simulink model "REMUS_CONTROL_helix"  (R2018a)
settings: Solver=FixedStepAuto  StartTime=0.0  StopTime=800  FixedStep=0.01  RelTol=1e-3  EnableMultiTasking=on
libraries: simulink x5, dspstat3 x1, simulink_extras x1
settings Model: Creator=wariza  LastModifiedBy=wariza
settings SolverCC: ZeroCrossControl=EnableAll  ZeroCrossAlgorithm=Adaptive  SolverResetMethod=Robust  PositivePriorityOrder=on  AutoInsertRateTranBlk=on  InsertRTBMode=Always
settings DataIOCC: LimitDataPoints=on  SaveFormat=Array
settings OptimizationCC: LifeSpan=inf
settings DebuggingCC: SolverPrmCheckMsg=warning  SFUnexpectedBacktrackingDiag=warning  SFNoUnconditionalDefaultTransitionDiag=warning  SFExecutionAtInitializationDiag=none
settings HardwareCC: ProdBitPerPointer=32  ProdBitPerSizeT=32  ProdBitPerPtrDiffT=32  ProdLargestAtomicFloat=None  ProdIntDivRoundTo=Undefined  ProdEndianess=Unspecified  ProdWordSize=32  ProdHWDeviceType=32-bit Generic
settings ModelReferenceCC: PropagateSignalLabelsOutOfModel=off
settings CodeAppCC: StateflowObjectComments=on
settings GRTTargetCC: TargetLangStandard=C89/C90 (ANSI)  GeneratePreprocessorConditionals=Disable all
settings ConfigComp: CovMetricSettings=dw  CovHtmlReporting=on  CovSaveCumulativeToWorkspaceVar=on  CovSaveSingleToWorkspaceVar=on  CovExternalEMLEnable=off  CovSFcnEnable=off

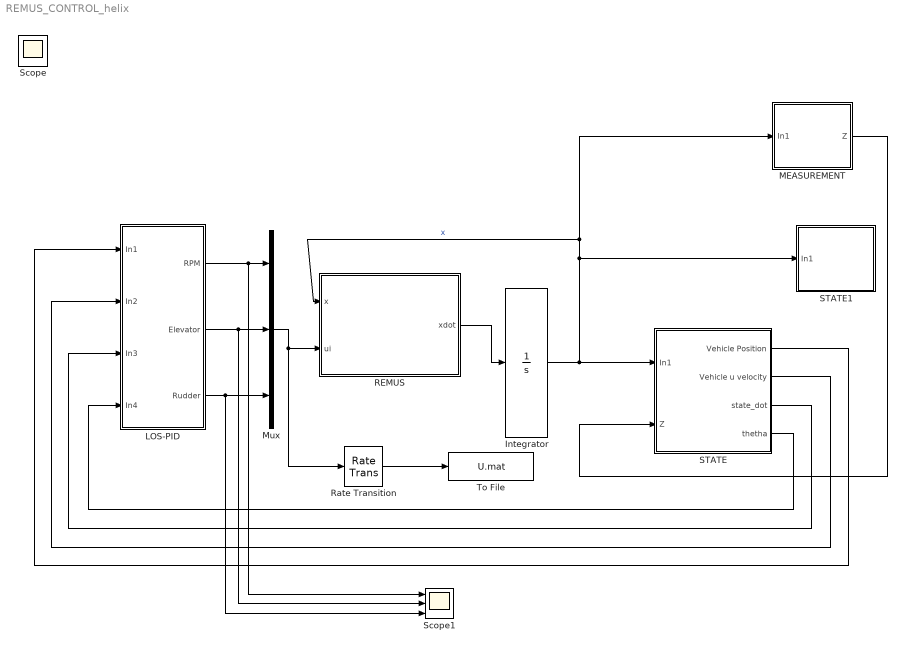
== system REMUS_CONTROL_helix ==
  Integrator : Integrator  InitialCondition=[0.5,0,0,0,0,0,60,3,0,0,0,3*pi/4]  ContinuousStateAttributes='position'
  LOS-PID : Subsystem
  MEASUREMENT : Subsystem
  Mux : Mux  Inputs=3
  REMUS : MATLAB Function  TreatAsAtomicUnit=on
  Rate Transition : RateTransition  OutPortSampleTime=0.01
  STATE : Subsystem
  STATE1 : Subsystem
  Scope1 : Scope  NumInputPorts=3
  To File : ToFile  Filename=U.mat  MatrixName=U
  Scope : Scope
  wires:
  Rate Transition/1 -> To File/1
  REMUS/1(xdot) -> Integrator/1
  Mux/1 -> Rate Transition/1, REMUS/2(ui)
  Integrator/1 -> STATE/1(In1), STATE1/1(In1), MEASUREMENT/1(In1), REMUS/1(x)  "x"
  MEASUREMENT/1(Z) -> STATE/2(Z)
  STATE/1(Vehicle Position) -> LOS-PID/1(In1)
  STATE/2(Vehicle u velocity) -> LOS-PID/2(In2)
  STATE/3(state_dot) -> LOS-PID/3(In3)
  STATE/4(thetha) -> LOS-PID/4(In4)
  LOS-PID/1(RPM) -> Scope1/1, Mux/1
  LOS-PID/2(Elevator) -> Scope1/2, Mux/2
  LOS-PID/3(Rudder) -> Scope1/3, Mux/3

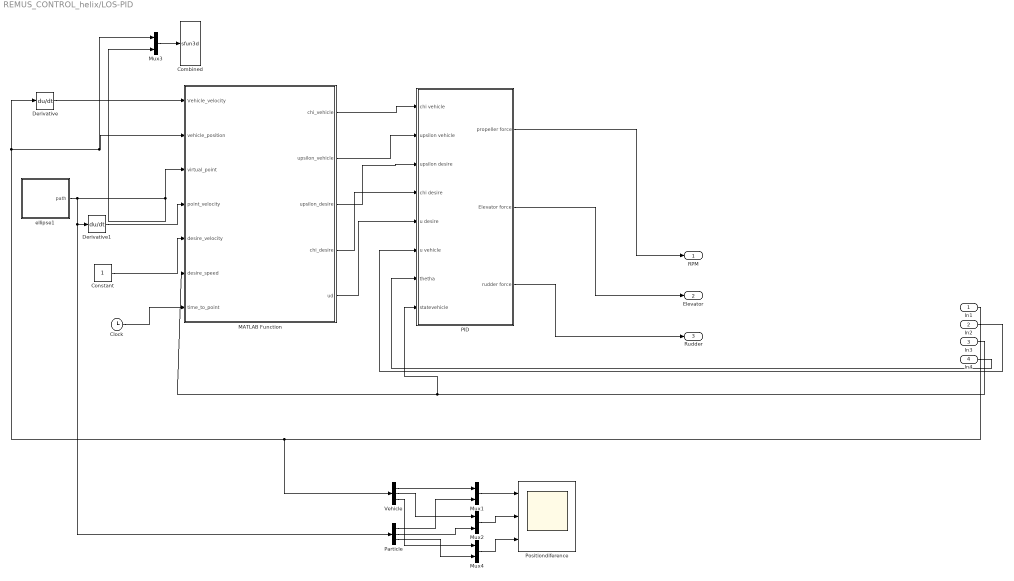
== system REMUS_CONTROL_helix/LOS-PID ==
  In1 : Inport
  In2 : Inport  Port=2
  In3 : Inport  Port=3
  In4 : Inport  Port=4
  Clock : Clock
  Combined : S-Function  LoadFcn=if exist('sfun3d','file'), sfun3d([],[],[],'LoadBlock'); end  FunctionName=sfun3d  Parameters=ax,T,np,cp,gd,ls,mk  SFunctionDeploymentMode=off  EnableBusSupport=off  mask(3D Graph){np=2, ax=[-100 100 -100 100 0 10], cp=[200 300 200], gd=on, ls=-, mk=none, T=-1}
      mask prompts: np "Number of point (lines)"; ax "[xmin xmax  ymin ymax zmin zmax]"; cp "Camera position (use [0 0 1] for 2D XY view)"; gd "Grid (on|off)"; ls "LineStyle"; mk "Marker"; T "Sampling Time"
      mask help:
      | This block plots the position of several points in the XYZ space. The input contains the coordinates of all the points (x1,y1,z1,x2,y2,z2,...).
      | The number of points (lines), the XYZ ranges, camera position, grid, linestyle, marker and sampling time, can be set as mask parameters.
      settings: CopyFcn=if exist('sfun3d','file'), sfun3d([],[],[],'CopyBlock'); end  DeleteFcn=if exist('sfun3d','file'), sfun3d([],[],[],'DeleteBlock'); end  NameChangeFcn=if exist('sfun3d','file'), sfun3d([],[],[],'NameChange'); end
      mask Help:
      | This block plots the position of several points in the XYZ space. The input contains the coordinates of all the points (x1,y1,z1,x2,y2,z2,...).
      | The number of points (lines), the XYZ ranges, camera position, grid, linestyle, marker and sampling time, can be set as mask parameters.
      mask TypeOptions ls: - | -- | : | -. | none
      mask TypeOptions mk: none | . | + | o | * | x | square | diamond | v | ^ | > | < | pentagram | hexagram
      mask Display: plot([.05 .95 .95 .05 .05],[.45 .45 .95 .95 .45], 0.5+cos(0:0.1:2*pi)*0.3,0.7+sin(0:0.1:2*pi)*0.2)
  Constant : Constant
  Derivative : Derivative
  Derivative1 : Derivative
  MATLAB Function : MATLAB Function  TreatAsAtomicUnit=on
  Mux{1..4} (4 alike) : Mux  Inputs=2
  PID : Subsystem
  Particle : Demux  Outputs=3
  Positiondiference : Scope  NumInputPorts=3
  Vehicle : Demux  Outputs=3
  ellipse1 : Subsystem
  RPM : Outport
  Elevator : Outport  Port=2
  Rudder : Outport  Port=3
  wires:
  Particle/2 -> Mux2/2
  Mux2/1 -> Positiondiference/2
  ellipse1/1(path) -> Derivative1/1, Particle/1, MATLAB Function/3(virtual_point), Mux3/2
  MATLAB Function/3(upsilon_desire) -> PID/3(upsilon desire)
  In4/1 -> PID/7(thetha)
  Particle/1 -> Mux1/2
  MATLAB Function/1(chi_vehicle) -> PID/1(chi vehicle)
  Mux3/1 -> Combined/1
  In1/1 -> Vehicle/1, Derivative/1, Mux3/1, MATLAB Function/2(vehicle_position)
  Mux1/1 -> Positiondiference/1
  MATLAB Function/2(upsilon_vehicle) -> PID/2(upsilon vehicle)
  Constant/1 -> MATLAB Function/5(desire_velocity)
  Mux4/1 -> Positiondiference/3
  PID/1(propeller force) -> RPM/1
  Clock/1 -> MATLAB Function/7(time_to_point)
  Derivative/1 -> MATLAB Function/1(Vehicle_velocity)
  Vehicle/2 -> Mux2/1
  Vehicle/3 -> Mux4/1
  Particle/3 -> Mux4/2
  PID/3(rudder force) -> Rudder/1
  MATLAB Function/5(ud) -> PID/5(u desire)
  In3/1 -> PID/8(statevehicle), MATLAB Function/6(desire_speed)
  Derivative1/1 -> MATLAB Function/4(point_velocity)
  MATLAB Function/4(chi_desire) -> PID/4(chi desire)
  Vehicle/1 -> Mux1/1
  In2/1 -> PID/6(u vehicle)
  PID/2(Elevator force) -> Elevator/1

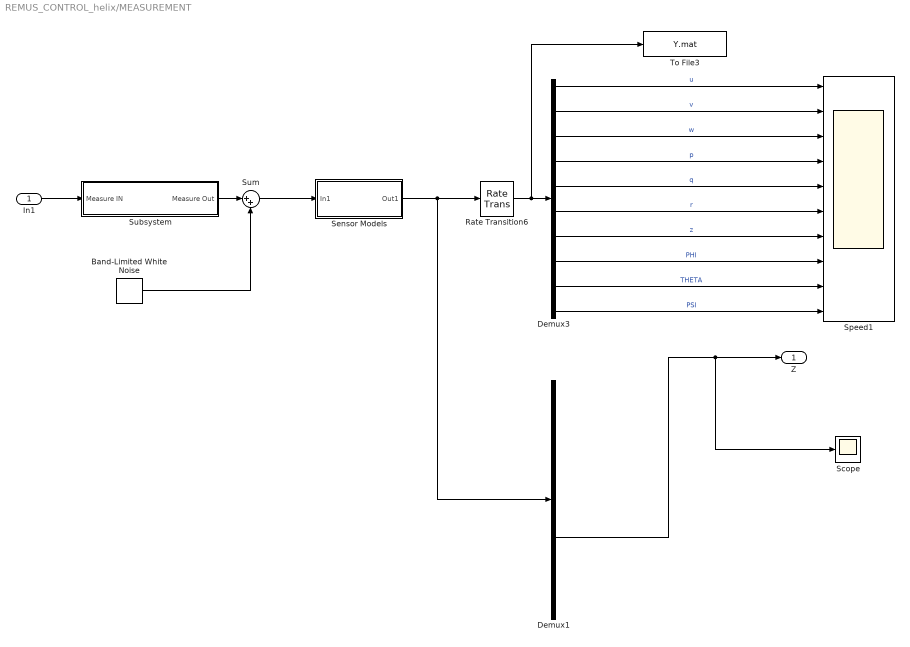
== system REMUS_CONTROL_helix/MEASUREMENT ==
  In1 : Inport
  Band-Limited White Noise : simulink/Sources/Band-Limited White Noise  Cov=[3e-8;2e-7;1e-8;1e-8;1e-7;1e-7;0.0000001;1e-9;1e-7;1e-5]  Ts=0.1  seed=[1;2;3;4;5;6;9;10;11;12]  VectorParams1D=off
  Demux1 : Demux  Outputs=10
  Demux3 : Demux  Outputs=10
  Rate Transition6 : RateTransition  OutPortSampleTime=0.01
  Scope : Scope
  Sensor Models : Subsystem
  Speed1 : Scope  NumInputPorts=10
  Subsystem : Subsystem
  Sum : Sum  Inputs=|++
  To File3 : ToFile  Filename=Y.mat  MatrixName=Y
  Z : Outport
  wires:
  Subsystem/1(Measure Out) -> Sum/1
  Demux3/3 -> Speed1/3  "w"
  Band-Limited White Noise/1 -> Sum/2
  Rate Transition6/1 -> To File3/1, Demux3/1
  Demux3/4 -> Speed1/4  "p"
  Demux3/2 -> Speed1/2  "v"
  Demux3/1 -> Speed1/1  "u"
  Sum/1 -> Sensor Models/1(In1)
  Demux3/5 -> Speed1/5  "q"
  Demux3/6 -> Speed1/6  "r"
  Demux3/9 -> Speed1/9  "THETA"
  Demux3/8 -> Speed1/8  "PHI"
  In1/1 -> Subsystem/1(Measure IN)
  Demux3/10 -> Speed1/10  "PSI"
  Demux3/7 -> Speed1/7  "z"
  Sensor Models/1(Out1) -> Demux1/1, Rate Transition6/1
  Demux1/7 -> Scope/1, Z/1

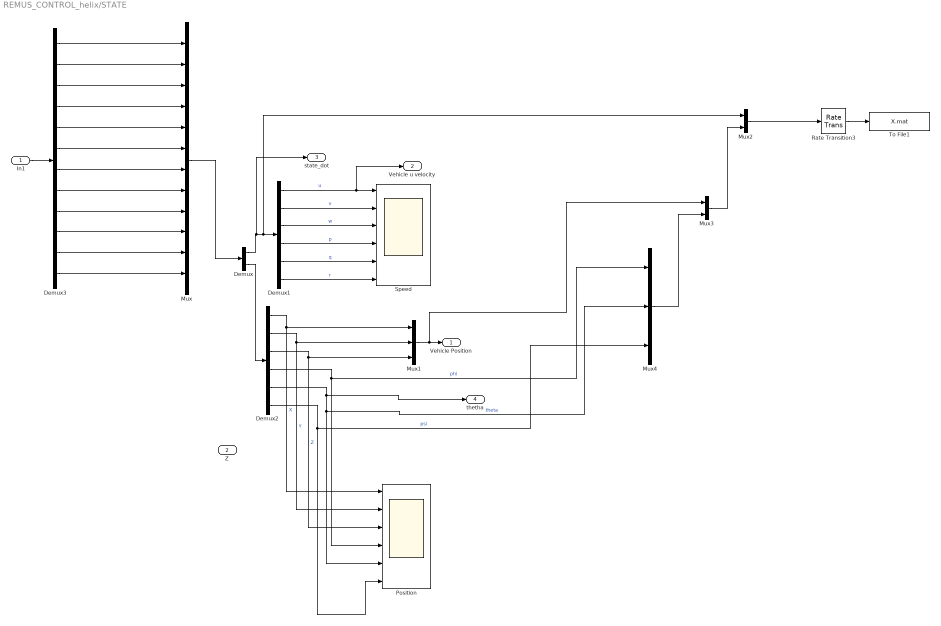
== system REMUS_CONTROL_helix/STATE ==
  In1 : Inport
  Z : Inport  Port=2
  Demux : Demux  Outputs=2
  Demux1 : Demux  Outputs=6
  Demux2 : Demux  Outputs=6
  Demux3 : Demux  Outputs=12
  Mux : Mux  Inputs=12
  Mux1 : Mux  Inputs=3
  Mux2 : Mux  Inputs=2
  Mux3 : Mux  Inputs=2
  Mux4 : Mux  Inputs=3
  Position : Scope  NumInputPorts=6
  Rate Transition3 : RateTransition  OutPortSampleTime=0.01
  Speed : Scope  NumInputPorts=6
  To File1 : ToFile  Filename=X.mat  MatrixName=X
  Vehicle Position : Outport
  Vehicle u velocity : Outport  Port=2
  state_dot : Outport  Port=3
  thetha : Outport  Port=4
  wires:
  Demux1/1 -> Vehicle u velocity/1, Speed/1  "u"
  Demux/2 -> Demux2/1
  Demux1/2 -> Speed/2  "v"
  Demux1/3 -> Speed/3  "w"
  Demux2/3 -> Mux1/3, Position/3  "Z"
  Demux2/5 -> thetha/1, Mux4/2, Position/5  "theta"
  Demux1/4 -> Speed/4  "p"
  Demux1/6 -> Speed/6  "r"
  Demux2/1 -> Mux1/1, Position/1  "X"
  Demux1/5 -> Speed/5  "q"
  Demux2/4 -> Mux4/1, Position/4  "phi"
  Demux2/2 -> Mux1/2, Position/2  "Y"
  Demux/1 -> state_dot/1, Mux2/1, Demux1/1
  Demux2/6 -> Mux4/3, Position/6  "psi"
  In1/1 -> Demux3/1
  Demux3/9 -> Mux/9
  Demux3/8 -> Mux/8
  Demux3/7 -> Mux/7
  Demux3/6 -> Mux/6
  Demux3/5 -> Mux/5
  Demux3/4 -> Mux/4
  Demux3/3 -> Mux/3
  Demux3/2 -> Mux/2
  Demux3/1 -> Mux/1
  Mux/1 -> Demux/1
  Mux1/1 -> Mux3/1, Vehicle Position/1
  Demux3/10 -> Mux/10
  Demux3/11 -> Mux/11
  Demux3/12 -> Mux/12
  Rate Transition3/1 -> To File1/1
  Mux2/1 -> Rate Transition3/1
  Mux4/1 -> Mux3/2
  Mux3/1 -> Mux2/2

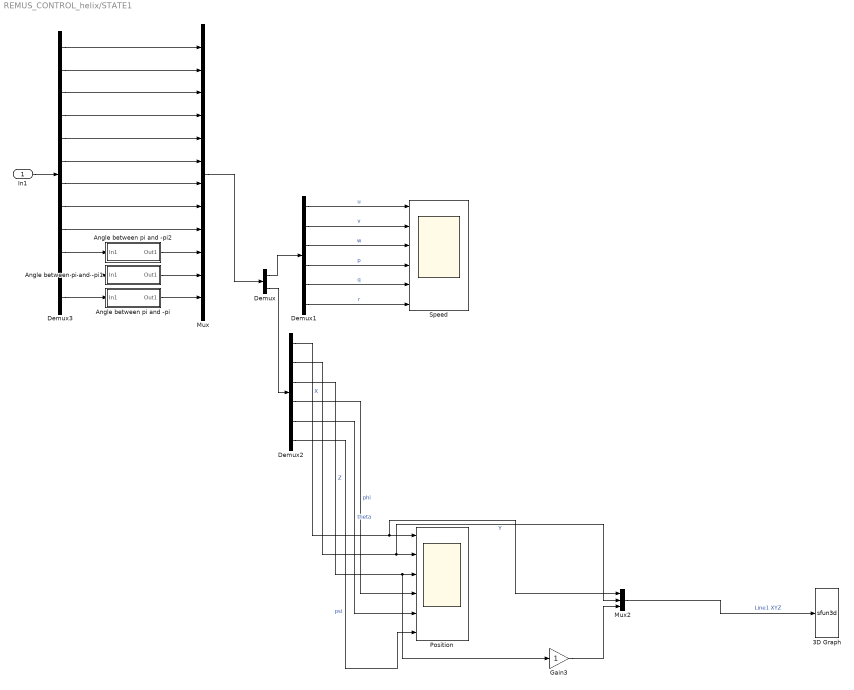
== system REMUS_CONTROL_helix/STATE1 ==
  In1 : Inport
  3D Graph : S-Function  LoadFcn=if exist('sfun3d','file'), sfun3d([],[],[],'LoadBlock'); end  FunctionName=sfun3d  Parameters=ax,T,np,cp,gd,ls,mk  SFunctionDeploymentMode=off  EnableBusSupport=off  mask(3D Graph){np=1, ax=[-100 100 -100 100 -30 30], cp=[20 40 20], gd=off, ls=-, mk=none, T=-1}
      mask prompts: np "Number of point (lines)"; ax "[xmin xmax  ymin ymax zmin zmax]"; cp "Camera position (use [0 0 1] for 2D XY view)"; gd "Grid (on|off)"; ls "LineStyle"; mk "Marker"; T "Sampling Time"
      mask help:
      | This block plots the position of several points in the XYZ space. The input contains the coordinates of all the points (x1,y1,z1,x2,y2,z2,...).
      | The number of points (lines), the XYZ ranges, camera position, grid, linestyle, marker and sampling time, can be set as mask parameters.
      settings: CopyFcn=if exist('sfun3d','file'), sfun3d([],[],[],'CopyBlock'); end  DeleteFcn=if exist('sfun3d','file'), sfun3d([],[],[],'DeleteBlock'); end  NameChangeFcn=if exist('sfun3d','file'), sfun3d([],[],[],'NameChange'); end
      mask Help:
      | This block plots the position of several points in the XYZ space. The input contains the coordinates of all the points (x1,y1,z1,x2,y2,z2,...).
      | The number of points (lines), the XYZ ranges, camera position, grid, linestyle, marker and sampling time, can be set as mask parameters.
      mask TypeOptions ls: - | -- | : | -. | none
      mask TypeOptions mk: none | . | + | o | * | x | square | diamond | v | ^ | > | < | pentagram | hexagram
      mask Display: plot([.05 .95 .95 .05 .05],[.45 .45 .95 .95 .45], 0.5+cos(0:0.1:2*pi)*0.3,0.7+sin(0:0.1:2*pi)*0.2)
  Angle between pi and -pi : Subsystem
  Angle between pi and -pi1 : Subsystem
  Angle between pi and -pi2 : Subsystem
  Demux : Demux  Outputs=2
  Demux1 : Demux  Outputs=6
  Demux2 : Demux  Outputs=6
  Demux3 : Demux  Outputs=12
  Gain3 : Gain
  Mux : Mux  Inputs=12
  Mux2 : Mux  Inputs=3
  Position : Scope  NumInputPorts=6
  Speed : Scope  NumInputPorts=6
  wires:
  Mux2/1 -> 3D Graph/1  "Line1 XYZ"
  Gain3/1 -> Mux2/3
  Demux1/1 -> Speed/1  "u"
  Demux/2 -> Demux2/1
  Demux1/2 -> Speed/2  "v"
  Demux1/3 -> Speed/3  "w"
  Demux2/3 -> Gain3/1, Position/3  "Z"
  Demux2/5 -> Position/5  "theta"
  Demux1/4 -> Speed/4  "p"
  Demux1/6 -> Speed/6  "r"
  Demux2/1 -> Mux2/1, Position/1  "X"
  Demux1/5 -> Speed/5  "q"
  Demux2/4 -> Position/4  "phi"
  Demux2/2 -> Mux2/2, Position/2  "Y"
  Demux/1 -> Demux1/1
  Demux2/6 -> Position/6  "psi"
  In1/1 -> Demux3/1
  Angle between pi and -pi/1(Out1) -> Mux/12
  Demux3/12 -> Angle between pi and -pi/1(In1)
  Angle between pi and -pi1/1(Out1) -> Mux/11
  Demux3/11 -> Angle between pi and -pi1/1(In1)
  Angle between pi and -pi2/1(Out1) -> Mux/10
  Demux3/10 -> Angle between pi and -pi2/1(In1)
  Demux3/9 -> Mux/9
  Demux3/8 -> Mux/8
  Demux3/7 -> Mux/7
  Demux3/6 -> Mux/6
  Demux3/5 -> Mux/5
  Demux3/4 -> Mux/4
  Demux3/3 -> Mux/3
  Demux3/2 -> Mux/2
  Demux3/1 -> Mux/1
  Mux/1 -> Demux/1

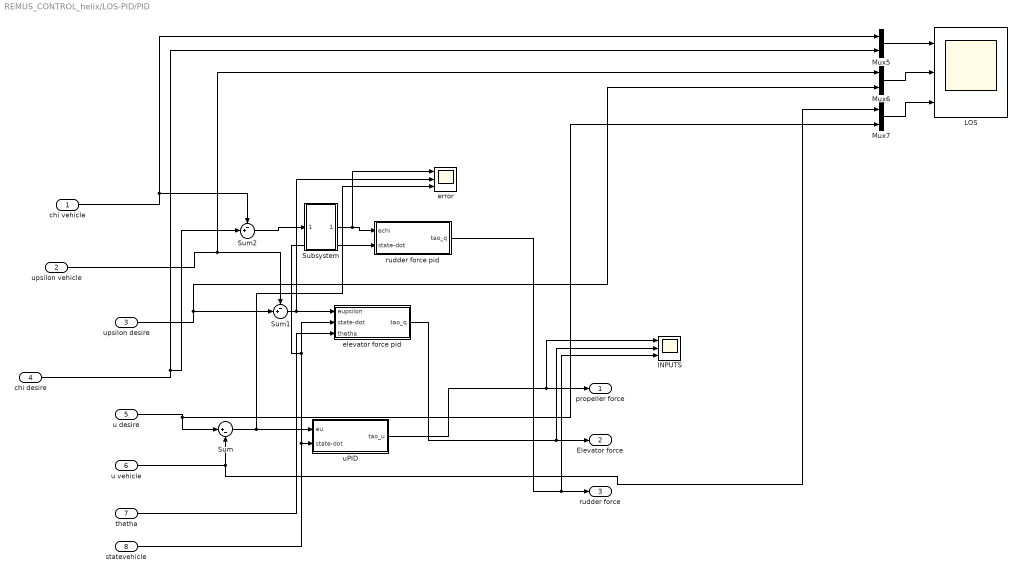
== system REMUS_CONTROL_helix/LOS-PID/PID ==
  chi vehicle : Inport
  upsilon vehicle : Inport  Port=2
  upsilon desire : Inport  Port=3
  chi desire : Inport  Port=4
  u desire : Inport  Port=5
  u vehicle : Inport  Port=6
  thetha : Inport  Port=7
  statevehicle : Inport  Port=8
  INPUTS : Scope  NumInputPorts=3
  LOS : Scope  NumInputPorts=3
  Mux5 : Mux  Inputs=2
  Mux6 : Mux  Inputs=2
  Mux7 : Mux  Inputs=2
  Subsystem : Subsystem
  Sum : Sum  Inputs=|+-
  Sum1 : Sum  Inputs=-+|
  Sum2 : Sum  Inputs=-+|
  elevator force pid : Subsystem
  error : Scope  NumInputPorts=3
  rudder force pid : Subsystem
  uPID : Subsystem
  propeller force : Outport
  Elevator force : Outport  Port=2
  rudder force : Outport  Port=3
  wires:
  uPID/1(tao_u) -> propeller force/1, INPUTS/1
  Mux6/1 -> LOS/2
  chi vehicle/1 -> Mux5/1, Sum2/1
  Sum/1 -> error/3, uPID/1(eu)
  statevehicle/1 -> rudder force pid/2(state-dot), elevator force pid/2(state-dot), uPID/2(state-dot)
  Sum1/1 -> error/2, elevator force pid/1(eupsilon)
  chi desire/1 -> Mux5/2, Sum2/2
  u vehicle/1 -> Mux7/1, Sum/2
  u desire/1 -> Sum/1, Mux7/2
  elevator force pid/1(tao_q) -> Elevator force/1, INPUTS/2
  rudder force pid/1(tao_q) -> rudder force/1, INPUTS/3
  upsilon desire/1 -> Mux6/2, Sum1/2
  Mux7/1 -> LOS/3
  thetha/1 -> elevator force pid/3(thetha)
  Mux5/1 -> LOS/1
  upsilon vehicle/1 -> Mux6/1, Sum1/1
  Sum2/1 -> Subsystem/1(In1)
  Subsystem/1(Out1) -> error/1, rudder force pid/1(echi)

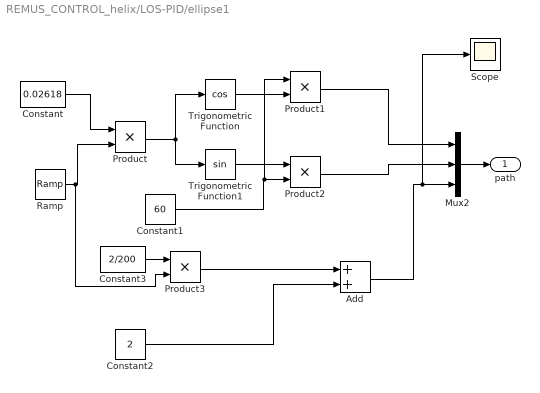
== system REMUS_CONTROL_helix/LOS-PID/ellipse1 ==
  Add : Sum
  Constant : Constant  Value=0.02618
  Constant1 : Constant  Value=60
  Constant2 : Constant  Value=2
  Constant3 : Constant  Value=2/200
  Mux2 : Mux  Inputs=3
  Product{,1..3} (4 alike) : Product
  Ramp : simulink/Sources/Ramp  slope=0.9  start=0  InitialOutput=0
  Scope : Scope
  Trigonometric Function : Trigonometry  Operator=cos
  Trigonometric Function1 : Trigonometry
  path : Outport
  wires:
  Mux2/1 -> path/1
  Ramp/1 -> Product3/2, Product/2
  Constant/1 -> Product/1
  Product/1 -> Trigonometric Function/1, Trigonometric Function1/1
  Trigonometric Function/1 -> Product1/2
  Trigonometric Function1/1 -> Product2/1
  Constant1/1 -> Product1/1, Product2/2
  Product1/1 -> Mux2/1
  Product2/1 -> Mux2/2
  Add/1 -> Scope/1, Mux2/3
  Constant2/1 -> Add/2
  Constant3/1 -> Product3/1
  Product3/1 -> Add/1

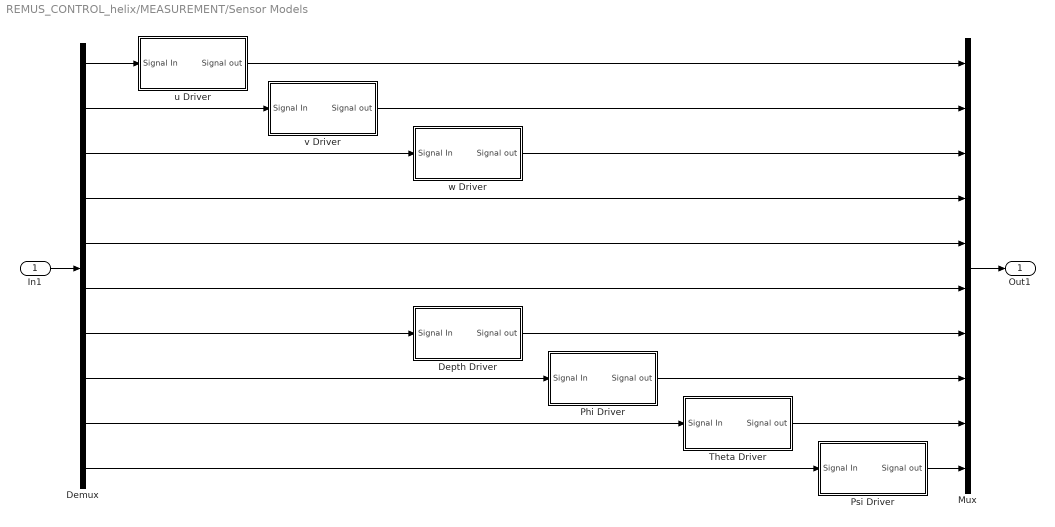
== system REMUS_CONTROL_helix/MEASUREMENT/Sensor Models ==
  In1 : Inport
  Demux : Demux  Outputs=10
  Depth Driver : Subsystem
  Mux : Mux  Inputs=10
  Phi Driver : Subsystem
  Psi Driver : Subsystem
  Theta Driver : Subsystem
  u Driver : Subsystem
  v Driver : Subsystem
  w Driver : Subsystem
  Out1 : Outport
  wires:
  In1/1 -> Demux/1
  Mux/1 -> Out1/1
  Demux/1 -> u Driver/1(Signal In)
  Demux/2 -> v Driver/1(Signal In)
  Demux/3 -> w Driver/1(Signal In)
  Demux/4 -> Mux/4
  Demux/5 -> Mux/5
  Demux/6 -> Mux/6
  Demux/8 -> Phi Driver/1(Signal In)
  Demux/9 -> Theta Driver/1(Signal In)
  Demux/10 -> Psi Driver/1(Signal In)
  Demux/7 -> Depth Driver/1(Signal In)
  Depth Driver/1(Signal out) -> Mux/7
  Phi Driver/1(Signal out) -> Mux/8
  Theta Driver/1(Signal out) -> Mux/9
  Psi Driver/1(Signal out) -> Mux/10
  u Driver/1(Signal out) -> Mux/1
  v Driver/1(Signal out) -> Mux/2
  w Driver/1(Signal out) -> Mux/3

== system REMUS_CONTROL_helix/MEASUREMENT/Subsystem ==
  note: u,v,w,p,q,r,Z,phi,theta,psi
  Measure IN : Inport
  Demux : Demux  Outputs=2
  Demux1 : Demux  Outputs=6
  Mux : Mux  Inputs=2
  Mux1 : Mux
  Measure Out : Outport
  wires:
  Measure IN/1 -> Demux/1
  Mux/1 -> Measure Out/1
  Demux/1 -> Mux/1
  Demux/2 -> Demux1/1
  Demux1/6 -> Mux1/4
  Demux1/5 -> Mux1/3
  Demux1/4 -> Mux1/2
  Demux1/3 -> Mux1/1
  Mux1/1 -> Mux/2

== system REMUS_CONTROL_helix/STATE1/Angle between pi and -pi ==
  In1 : Inport
  Atan2 : Trigonometry  Operator=atan2
  Cos : Trigonometry
  Sin : Trigonometry  Operator=cos
  Out1 : Outport
  wires:
  Cos/1 -> Atan2/1
  In1/1 -> Cos/1, Sin/1
  Sin/1 -> Atan2/2
  Atan2/1 -> Out1/1

== system REMUS_CONTROL_helix/STATE1/Angle between pi and -pi1 ==
  In1 : Inport
  Atan2 : Trigonometry  Operator=atan2
  Cos : Trigonometry
  Sin : Trigonometry  Operator=cos
  Out1 : Outport
  wires:
  Cos/1 -> Atan2/1
  In1/1 -> Cos/1, Sin/1
  Sin/1 -> Atan2/2
  Atan2/1 -> Out1/1

== system REMUS_CONTROL_helix/STATE1/Angle between pi and -pi2 ==
  In1 : Inport
  Atan2 : Trigonometry  Operator=atan2
  Cos : Trigonometry
  Sin : Trigonometry  Operator=cos
  Out1 : Outport
  wires:
  Cos/1 -> Atan2/1
  In1/1 -> Cos/1, Sin/1
  Sin/1 -> Atan2/2
  Atan2/1 -> Out1/1

== system REMUS_CONTROL_helix/LOS-PID/PID/Subsystem ==
  In1 : Inport
  Trigonometric Function : Trigonometry
  Trigonometric Function1 : Trigonometry  Operator=cos
  Trigonometric Function2 : Trigonometry  Operator=atan2
  Out1 : Outport
  wires:
  Trigonometric Function/1 -> Trigonometric Function2/1
  Trigonometric Function2/1 -> Out1/1
  In1/1 -> Trigonometric Function1/1, Trigonometric Function/1
  Trigonometric Function1/1 -> Trigonometric Function2/2

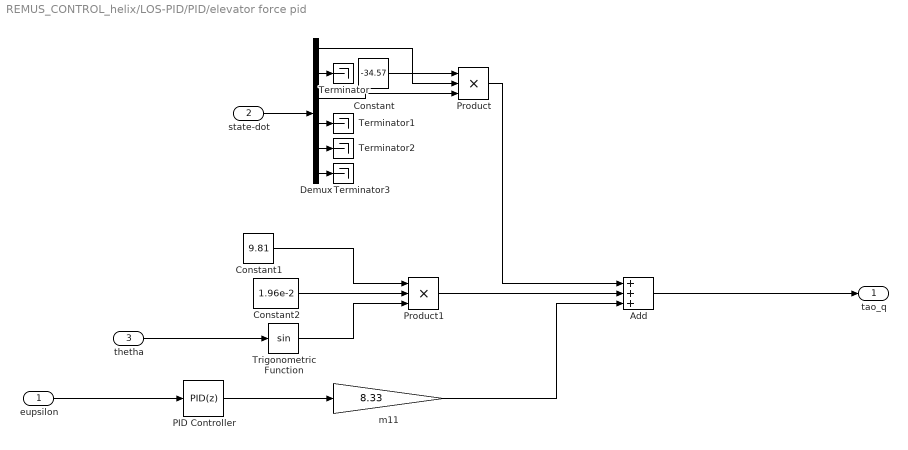
== system REMUS_CONTROL_helix/LOS-PID/PID/elevator force pid ==
  eupsilon : Inport
  state-dot : Inport  Port=2
  thetha : Inport  Port=3
  Add : Sum  Inputs=+++
  Constant : Constant  Value=-34.57
  Constant1 : Constant  Value=9.81
  Constant2 : Constant  Value=1.96e-2
  Demux : Demux  Outputs=6
  PID Controller : simulink/Continuous/PID Controller  Controller=PID  TimeDomain=Discrete-time  SampleTime=.4  IntegratorMethod=Forward Euler  FilterMethod=Forward Euler  Form=Parallel  UseFilter=off  ControllerParametersSource=internal  P=2  I=0  D=0.5  N=100  InitialConditionSource=internal  InitialConditionForIntegrator=0  InitialConditionForFilter=0  ExternalReset=none  LimitOutput=off  UpperSaturationLimit=inf  LowerSaturationLimit=-inf  LinearizeAsGain=on  AntiWindupMode=none  Kb=1  TrackingMode=off  Kt=1  PParamMin=[]  PParamMax=[]  IParamMin=[]  IParamMax=[]  DParamMin=[]  DParamMax=[]  NParamMin=[]  NParamMax=[]  KbParamMin=[]  KbParamMax=[]  KtParamMin=[]  KtParamMax=[]  POutMin=[]  POutMax=[]  IOutMin=[]  IOutMax=[]  DOutMin=[]  DOutMax=[]  NOutMin=[]  NOutMax=[]  KbOutMin=[]  KbOutMax=[]  KtOutMin=[]  KtOutMax=[]  IntegratorOutMin=[]  IntegratorOutMax=[]  FilterOutMin=[]  FilterOutMax=[]  SumOutMin=[]  SumOutMax=[]  SumI1OutMin=[]  SumI1OutMax=[]  SumI2OutMin=[]  SumI2OutMax=[]  SumI3OutMin=[]  SumI3OutMax=[]  SumDOutMin=[]  SumDOutMax=[]  SaturationOutMin=[]  SaturationOutMax=[]  IntegratorContinuousStateAttributes=''  IntegratorStateMustResolveToSignalObject=off  IntegratorRTWStateStorageClass=Auto  FilterContinuousStateAttributes=''  FilterStateMustResolveToSignalObject=off  FilterRTWStateStorageClass=Auto  DifferentiatorICPrevScaledInput=0  DifferentiatorOutMin=[]  DifferentiatorOutMax=[]  FilterDiffOutCoefMin=[]  FilterDiffOutCoefMax=[]  SumDenOutMin=[]  SumDenOutMax=[]  SumNumOutMin=[]  SumNumOutMax=[]  ReciprocalOutMin=[]  ReciprocalOutMax=[]  DivideOutMin=[]  DivideOutMax=[]  TunerSelectOption=Transfer Function Based (PID Tuner App)
  Product : Product  Inputs=3
  Product1 : Product  Inputs=3
  Terminator{,1..3} (4 alike) : Terminator
  Trigonometric Function : Trigonometry
  m11 : Gain  Gain=8.33
  tao_q : Outport  InitialOutput=0
  wires:
  state-dot/1 -> Demux/1
  Constant/1 -> Product/1
  m11/1 -> Add/3
  Constant1/1 -> Product1/1
  Demux/1 -> Product/2
  Demux/3 -> Product/3
  Product/1 -> Add/1
  Constant2/1 -> Product1/2
  Trigonometric Function/1 -> Product1/3
  Product1/1 -> Add/2
  thetha/1 -> Trigonometric Function/1
  PID Controller/1 -> m11/1
  eupsilon/1 -> PID Controller/1
  Add/1 -> tao_q/1
  Demux/6 -> Terminator3/1
  Demux/5 -> Terminator2/1
  Demux/4 -> Terminator1/1
  Demux/2 -> Terminator/1

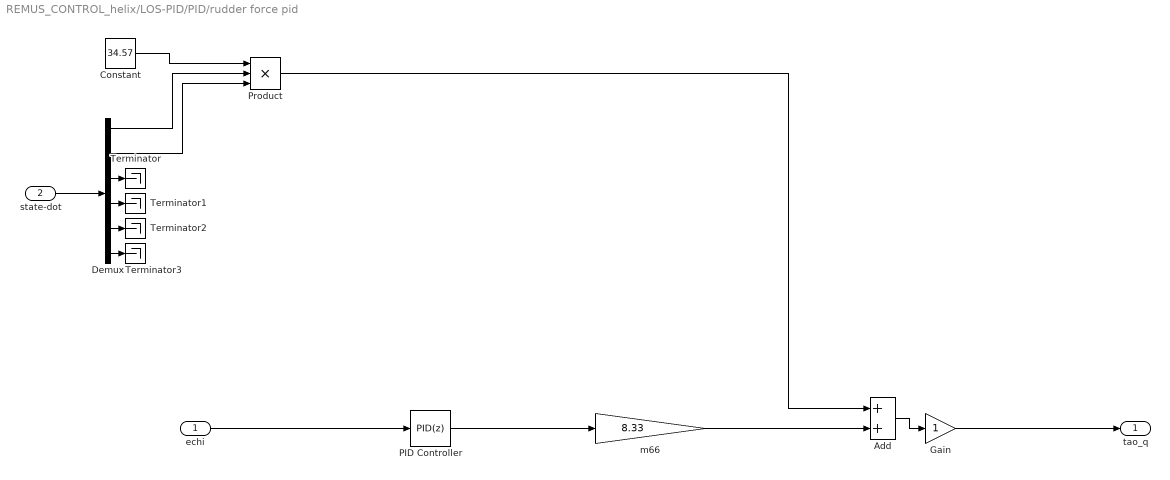
== system REMUS_CONTROL_helix/LOS-PID/PID/rudder force pid ==
  echi : Inport
  state-dot : Inport  Port=2
  Add : Sum
  Constant : Constant  Value=34.57
  Demux : Demux  Outputs=6
  Gain : Gain
  PID Controller : simulink/Continuous/PID Controller  Controller=PID  TimeDomain=Discrete-time  SampleTime=0.4  IntegratorMethod=Forward Euler  FilterMethod=Forward Euler  Form=Parallel  UseFilter=off  ControllerParametersSource=internal  P=3  I=0  D=1  N=100  InitialConditionSource=internal  InitialConditionForIntegrator=0  InitialConditionForFilter=0  ExternalReset=none  LimitOutput=on  UpperSaturationLimit=inf  LowerSaturationLimit=-inf  LinearizeAsGain=on  AntiWindupMode=clamping  Kb=1  TrackingMode=off  Kt=1  PParamMin=[]  PParamMax=[]  IParamMin=[]  IParamMax=[]  DParamMin=[]  DParamMax=[]  NParamMin=[]  NParamMax=[]  KbParamMin=[]  KbParamMax=[]  KtParamMin=[]  KtParamMax=[]  POutMin=[]  POutMax=[]  IOutMin=[]  IOutMax=[]  DOutMin=[]  DOutMax=[]  NOutMin=[]  NOutMax=[]  KbOutMin=[]  KbOutMax=[]  KtOutMin=[]  KtOutMax=[]  IntegratorOutMin=[]  IntegratorOutMax=[]  FilterOutMin=[]  FilterOutMax=[]  SumOutMin=[]  SumOutMax=[]  SumI1OutMin=[]  SumI1OutMax=[]  SumI2OutMin=[]  SumI2OutMax=[]  SumI3OutMin=[]  SumI3OutMax=[]  SumDOutMin=[]  SumDOutMax=[]  SaturationOutMin=[]  SaturationOutMax=[]  IntegratorContinuousStateAttributes=''  IntegratorStateMustResolveToSignalObject=off  IntegratorRTWStateStorageClass=Auto  FilterContinuousStateAttributes=''  FilterStateMustResolveToSignalObject=off  FilterRTWStateStorageClass=Auto  DifferentiatorICPrevScaledInput=0  DifferentiatorOutMin=[]  DifferentiatorOutMax=[]  FilterDiffOutCoefMin=[]  FilterDiffOutCoefMax=[]  SumDenOutMin=[]  SumDenOutMax=[]  SumNumOutMin=[]  SumNumOutMax=[]  ReciprocalOutMin=[]  ReciprocalOutMax=[]  DivideOutMin=[]  DivideOutMax=[]  TunerSelectOption=Transfer Function Based (PID Tuner App)
  Product : Product  Inputs=3
  Terminator{,1..3} (4 alike) : Terminator
  m66 : Gain  Gain=8.33
  tao_q : Outport  InitialOutput=0
  wires:
  state-dot/1 -> Demux/1
  Constant/1 -> Product/1
  m66/1 -> Add/2
  Demux/1 -> Product/2
  Product/1 -> Add/1
  Demux/2 -> Product/3
  Add/1 -> Gain/1
  PID Controller/1 -> m66/1
  Gain/1 -> tao_q/1
  Demux/6 -> Terminator3/1
  Demux/5 -> Terminator2/1
  Demux/4 -> Terminator1/1
  Demux/3 -> Terminator/1
  echi/1 -> PID Controller/1

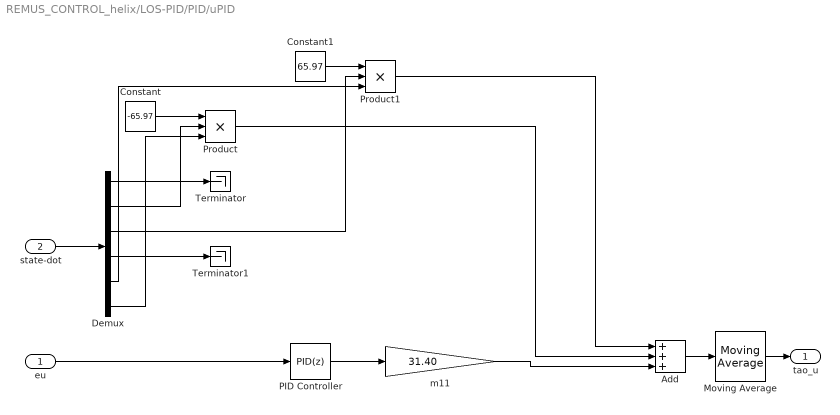
== system REMUS_CONTROL_helix/LOS-PID/PID/uPID ==
  eu : Inport
  state-dot : Inport  Port=2
  Add : Sum  Inputs=+++
  Constant : Constant  Value=-65.97
  Constant1 : Constant  Value=65.97
  Demux : Demux  Outputs=6
  Moving Average : dspstat3/Moving Average  Method=Exponential weighting  ForgettingFactorPort=off  SpecifyWindowLength=on  WindowLength=20  ForgettingFactor=0.9  SimulateUsing=Code generation
  PID Controller : simulink/Continuous/PID Controller  Controller=PID  TimeDomain=Discrete-time  SampleTime=0.4  IntegratorMethod=Forward Euler  FilterMethod=Forward Euler  Form=Parallel  UseFilter=off  ControllerParametersSource=internal  P=100  I=1  D=2  N=50  InitialConditionSource=internal  InitialConditionForIntegrator=0  InitialConditionForFilter=0  ExternalReset=none  ZeroCross=off  LimitOutput=off  UpperSaturationLimit=inf  LowerSaturationLimit=-inf  LinearizeAsGain=on  AntiWindupMode=none  Kb=1  TrackingMode=off  Kt=1  PParamMin=[]  PParamMax=[]  IParamMin=[]  IParamMax=[]  DParamMin=[]  DParamMax=[]  NParamMin=[]  NParamMax=[]  KbParamMin=[]  KbParamMax=[]  KtParamMin=[]  KtParamMax=[]  POutMin=[]  POutMax=[]  IOutMin=[]  IOutMax=[]  DOutMin=[]  DOutMax=[]  NOutMin=[]  NOutMax=[]  KbOutMin=[]  KbOutMax=[]  KtOutMin=[]  KtOutMax=[]  IntegratorOutMin=[]  IntegratorOutMax=[]  FilterOutMin=[]  FilterOutMax=[]  SumOutMin=[]  SumOutMax=[]  SumI1OutMin=[]  SumI1OutMax=[]  SumI2OutMin=[]  SumI2OutMax=[]  SumI3OutMin=[]  SumI3OutMax=[]  SumDOutMin=[]  SumDOutMax=[]  SaturationOutMin=[]  SaturationOutMax=[]  IntegratorContinuousStateAttributes=''  IntegratorStateMustResolveToSignalObject=off  IntegratorRTWStateStorageClass=Auto  FilterContinuousStateAttributes=''  FilterStateMustResolveToSignalObject=off  FilterRTWStateStorageClass=Auto  DifferentiatorICPrevScaledInput=0  DifferentiatorOutMin=[]  DifferentiatorOutMax=[]  FilterDiffOutCoefMin=[]  FilterDiffOutCoefMax=[]  SumDenOutMin=[]  SumDenOutMax=[]  SumNumOutMin=[]  SumNumOutMax=[]  ReciprocalOutMin=[]  ReciprocalOutMax=[]  DivideOutMin=[]  DivideOutMax=[]  TunerSelectOption=Transfer Function Based (PID Tuner App)
  Product : Product  Inputs=3
  Product1 : Product  Inputs=3
  Terminator : Terminator
  Terminator1 : Terminator
  m11 : Gain  Gain=31.40
  tao_u : Outport  InitialOutput=0
  wires:
  eu/1 -> PID Controller/1
  PID Controller/1 -> m11/1
  state-dot/1 -> Demux/1
  Constant/1 -> Product/1
  Demux/2 -> Product/2
  m11/1 -> Add/3
  Product/1 -> Add/2
  Demux/6 -> Product/3
  Constant1/1 -> Product1/1
  Demux/3 -> Product1/2
  Demux/5 -> Product1/3
  Product1/1 -> Add/1
  Add/1 -> Moving Average/1
  Moving Average/1 -> tao_u/1
  Demux/4 -> Terminator1/1
  Demux/1 -> Terminator/1

== system REMUS_CONTROL_helix/MEASUREMENT/Sensor Models/Depth Driver ==
  Signal In : Inport
  Constant : Constant  Value=2^14/100
  Constant1 : Constant  Value=100/2^14
  Mux1 : Mux  Inputs=2
  Product : Product
  Product1 : Product
  Rounding Function : Rounding  Operator=round
  Saturation : Saturate  UpperLimit=100  LowerLimit=-100
  Scope : Scope
  Signal out : Outport
  wires:
  Signal In/1 -> Mux1/2, Product/1
  Constant/1 -> Product/2
  Mux1/1 -> Scope/1
  Saturation/1 -> Signal out/1, Mux1/1
  Constant1/1 -> Product1/2
  Product1/1 -> Saturation/1
  Rounding Function/1 -> Product1/1
  Product/1 -> Rounding Function/1

== system REMUS_CONTROL_helix/MEASUREMENT/Sensor Models/Phi Driver ==
  Signal In : Inport
  Angle between pi and -pi : Subsystem
  Constant : Constant  Value=2^14/(2*pi)
  Constant1 : Constant  Value=2*pi/2^14
  Mux1 : Mux  Inputs=2
  Product : Product
  Product1 : Product
  Rounding Function : Rounding  Operator=round
  Scope : Scope
  Signal out : Outport
  wires:
  Signal In/1 -> Mux1/2, Product/1
  Constant/1 -> Product/2
  Mux1/1 -> Scope/1
  Constant1/1 -> Product1/2
  Rounding Function/1 -> Product1/1
  Product1/1 -> Angle between pi and -pi/1(In1)
  Product/1 -> Rounding Function/1
  Angle between pi and -pi/1(Out1) -> Signal out/1, Mux1/1

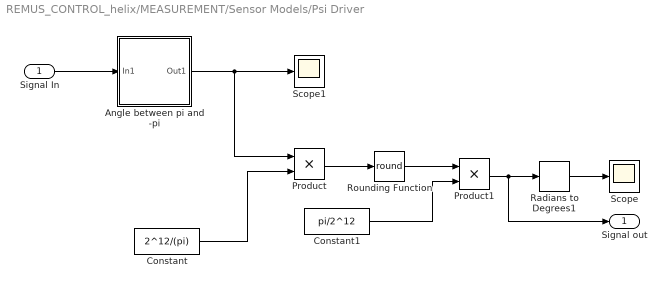
== system REMUS_CONTROL_helix/MEASUREMENT/Sensor Models/Psi Driver ==
  Signal In : Inport
  Angle between pi and -pi : Subsystem
  Constant : Constant  Value=2^12/(pi)
  Constant1 : Constant  Value=pi/2^12
  Product : Product
  Product1 : Product
  Radians to Degrees1 : simulink_extras/Transformations/Radians to Degrees
  Rounding Function : Rounding  Operator=round
  Scope : Scope
  Scope1 : Scope
  Signal out : Outport
  wires:
  Constant/1 -> Product/2
  Radians to Degrees1/1 -> Scope/1
  Constant1/1 -> Product1/2
  Rounding Function/1 -> Product1/1
  Product/1 -> Rounding Function/1
  Product1/1 -> Signal out/1, Radians to Degrees1/1
  Signal In/1 -> Angle between pi and -pi/1(In1)
  Angle between pi and -pi/1(Out1) -> Product/1, Scope1/1

== system REMUS_CONTROL_helix/MEASUREMENT/Sensor Models/Theta Driver ==
  Signal In : Inport
  Angle between pi and -pi : Subsystem
  Constant : Constant  Value=2^12/(2*pi)
  Constant1 : Constant  Value=2*pi/2^12
  Mux1 : Mux  Inputs=2
  Product : Product
  Product1 : Product
  Rounding Function : Rounding  Operator=round
  Scope : Scope
  Signal out : Outport
  wires:
  Signal In/1 -> Mux1/2, Product/1
  Constant/1 -> Product/2
  Mux1/1 -> Scope/1
  Constant1/1 -> Product1/2
  Rounding Function/1 -> Product1/1
  Product1/1 -> Angle between pi and -pi/1(In1)
  Product/1 -> Rounding Function/1
  Angle between pi and -pi/1(Out1) -> Signal out/1, Mux1/1

== system REMUS_CONTROL_helix/MEASUREMENT/Sensor Models/u Driver ==
  Signal In : Inport
  Constant : Constant  Value=2^12/4
  Constant1 : Constant  Value=4/2^12
  Mux1 : Mux  Inputs=2
  Product : Product
  Product1 : Product
  Rounding Function : Rounding  Operator=round
  Saturation : Saturate  UpperLimit=3  LowerLimit=-1
  Scope : Scope
  Signal out : Outport
  wires:
  Signal In/1 -> Mux1/2, Product/1
  Constant/1 -> Product/2
  Mux1/1 -> Scope/1
  Saturation/1 -> Signal out/1, Mux1/1
  Constant1/1 -> Product1/2
  Product1/1 -> Saturation/1
  Rounding Function/1 -> Product1/1
  Product/1 -> Rounding Function/1

== system REMUS_CONTROL_helix/MEASUREMENT/Sensor Models/v Driver ==
  Signal In : Inport
  Constant : Constant  Value=2^12/4
  Constant1 : Constant  Value=4/2^12
  Mux1 : Mux  Inputs=2
  Product : Product
  Product1 : Product
  Rounding Function : Rounding  Operator=round
  Saturation : Saturate  UpperLimit=3  LowerLimit=-1
  Scope : Scope
  Signal out : Outport
  wires:
  Signal In/1 -> Mux1/2, Product/1
  Constant/1 -> Product/2
  Mux1/1 -> Scope/1
  Saturation/1 -> Signal out/1, Mux1/1
  Constant1/1 -> Product1/2
  Product1/1 -> Saturation/1
  Rounding Function/1 -> Product1/1
  Product/1 -> Rounding Function/1

== system REMUS_CONTROL_helix/MEASUREMENT/Sensor Models/w Driver ==
  Signal In : Inport
  Constant : Constant  Value=2^12/4
  Constant1 : Constant  Value=4/2^12
  Mux1 : Mux  Inputs=2
  Product : Product
  Product1 : Product
  Rounding Function : Rounding  Operator=round
  Saturation : Saturate  UpperLimit=3  LowerLimit=-1
  Scope : Scope
  Signal out : Outport
  wires:
  Signal In/1 -> Mux1/2, Product/1
  Constant/1 -> Product/2
  Mux1/1 -> Scope/1
  Saturation/1 -> Signal out/1, Mux1/1
  Constant1/1 -> Product1/2
  Product1/1 -> Saturation/1
  Rounding Function/1 -> Product1/1
  Product/1 -> Rounding Function/1

== system REMUS_CONTROL_helix/MEASUREMENT/Sensor Models/Phi Driver/Angle between pi and -pi ==
  In1 : Inport
  Atan2 : Trigonometry  Operator=atan2
  Cos : Trigonometry
  Sin : Trigonometry  Operator=cos
  Out1 : Outport
  wires:
  Cos/1 -> Atan2/1
  In1/1 -> Cos/1, Sin/1
  Sin/1 -> Atan2/2
  Atan2/1 -> Out1/1

== system REMUS_CONTROL_helix/MEASUREMENT/Sensor Models/Psi Driver/Angle between pi and -pi ==
  In1 : Inport
  Atan2 : Trigonometry  Operator=atan2
  Cos : Trigonometry
  Sin : Trigonometry  Operator=cos
  Out1 : Outport
  wires:
  Cos/1 -> Atan2/1
  In1/1 -> Cos/1, Sin/1
  Sin/1 -> Atan2/2
  Atan2/1 -> Out1/1

== system REMUS_CONTROL_helix/MEASUREMENT/Sensor Models/Theta Driver/Angle between pi and -pi ==
  In1 : Inport
  Atan2 : Trigonometry  Operator=atan2
  Cos : Trigonometry
  Sin : Trigonometry  Operator=cos
  Out1 : Outport
  wires:
  Cos/1 -> Atan2/1
  In1/1 -> Cos/1, Sin/1
  Sin/1 -> Atan2/2
  Atan2/1 -> Out1/1

== matlab function REMUS_CONTROL_helix/LOS-PID/MATLAB Function ==
  data: Vehicle_velocity input; chi_vehicle output; vehicle_position input; virtual_point input; point_velocity input; desire_velocity input; upsilon_vehicle output; upsilon_desire output; chi_desire output; ud output; desire_speed input; time_to_point input
function [chi_vehicle,upsilon_vehicle,upsilon_desire,chi_desire,ud]=LOS(Vehicle_velocity,vehicle_position,virtual_point,point_velocity,desire_velocity,desire_speed,time_to_point)
% Vehicle_velocity: vehicle vector of velocity [x_dot,y_dot,z_dot]
% vehicle_position: position vector[X,Y,Z]
% virtual_point; virtual point position vector[X,Y,Z]
% time_to_point= step time
%desire speed vector [u,v,w]
%desire_velocity Ud
chi_vehicle=0;
upsilon_vehicle=0;
upsilon_desire=0;
chi_desire=0;
ud=0;
% orientation vehicle asimuth and elevation
chi_vehicle=atan2(Vehicle_velocity(2),Vehicle_velocity(1));

if chi_vehicle< pi
    chi_vehicle = chi_vehicle;
else
    chi_vehicle = chi_vehicle-pi;
end
if Vehicle_velocity==[0,0,0]'
    upsilon_vehicle=atan(0);
else
upsilon_vehicle=atan(-Vehicle_velocity(3)/sqrt(Vehicle_velocity(2)^2+Vehicle_velocity(1)^2));
end
% orientation point
virtual_point_velocity=point_velocity;
% if time_to_point==0
%     virtual_point_velocity=[0,0,0]' ;
%     psi_point=0;
%     theta_point=0;
% else
    psi_point=atan2(virtual_point_velocity(2),virtual_point_velocity(1));
    theta_point=atan(-virtual_point_velocity(3)/sqrt(virtual_point_velocity(2)^2+virtual_point_velocity(1)^2));
% end

x=vehicle_position(1);
y=vehicle_position(2);
z=vehicle_position(3);
x_p=virtual_point(1);
y_p=virtual_point(2);
z_p=virtual_point(3);
% error vector
x_e=cos(psi_point)*cos(theta_point)*(x-x_p)+sin(psi_point)*cos(theta_point)*(y-y_p)-sin(theta_point)*(z-z_p);
y_e=-sin(psi_point)*(x-x_p)+cos(psi_point)*(y-y_p);
z_e=cos(psi_point)*sin(theta_point)*(x-x_p)+sin(psi_point)*sin(theta_point)*(y-y_p)+cos(theta_point)*(z-z_p);

% LOS Guidance angles
ky=1;
kz=1;
deltay=150;
deltaz=50;
psi_r=tanh(-ky*y_e/deltay);
theta_r=tanh(kz*z_e/deltaz);
u=desire_speed(1);
v=desire_speed(2);
w=desire_speed(3);

% Guidance Law
upsilon_desire=asin(sin(theta_point)*cos(theta_r)*cos(psi_r)+cos(theta_point)*sin(theta_r));
chi_y=cos(psi_point)*sin(psi_r)*cos(theta_r)-sin(theta_point)*sin(theta_r)*sin(psi_point)+sin(psi_point)*cos(psi_r)*cos(theta_point)*cos(theta_r);
chi_x=-sin(psi_point)*sin(psi_r)*cos(theta_r)-sin(theta_point)*sin(theta_r)*cos(psi_point)+cos(psi_point)*cos(psi_r)*cos(theta_point)*cos(theta_r);
chi_desire=atan2(chi_y,chi_x);
if time_to_point==0
    chi_desire=0;
    upsilon_desire=0;
end





% % k=1;

if time_to_point==0
  
else
    desire_velocity=(norm(virtual_point_velocity)-0.05*x_e)/(cos(psi_r)*cos(theta_r));
end

if desire_velocity>=2.5
    desire_velocity=2.5;
end
if desire_velocity<=0
    desire_velocity=0;
end
ud=desire_velocity*u/sqrt(u^2+v^2+w^2);
a=isnan(ud);

end

== matlab function REMUS_CONTROL_helix/REMUS ==
  data: x input; xdot output double; ui input
function xdot= REMUS(x,ui)
% Simulation algorithm for REMUS This code is based in:
% Prestero, T., 2001. Verification of a six-degree of freedom simulation 
% model for the REMUS autonomous underwater vehicle (Doctoral dissertation, 
% Massachusetts Institute of Technology and Woods Hole Oceanographic 
% Institution).         
            
%              _____F1__________________________________
%          |  /           ||                       ||   \
%          |==      F3    ||       Remus           ||    | 
%          |  \___________||_______________________||___/
%                   F2
% V=[u,v,w,p,q,r,x,y,z,phi,psi,theta];


% TERMS
% ---------------------------------------------
%STATE VECTOR:
%
% x = (u v w p q r xpos ypos zpos phi theta psi) ,
% Body-referenced Coordinates
% u  = Surge velocity [m/s]
% v  = Sway velocity  [m/s]
% w  = Heave velocity [m/s]
% p  = Roll rate      [rad/s]
% q  = Pitch rate     [rad/s]
% r  = Yaw rate       [rad/s]
%
% Earth-fixed coordinates
% xpos  = Position in x-direction [m]
% ypos  = Position in y-direction [m]
% zpos  = Position in z-direction [m]
% phi   = Roll angle              [rad]
% theta = Pitch angle             [rad]
% psi   = Yaw angle               [rad]
%
%INPUT VECTOR
% ui = [n delta_s delta_r]'
%  Control Fin Angles
%   n= shaft speed RPM
%   delta_s = angle of stern planes  [rad]
%   delta_r = angle of rudder planes [rad]

% Get state variables
u     = x(1); 
v     = x(2); 
w     = x(3); 
p     = x(4); 
q     = x(5); 
r     = x(6);
phi   = x(10); 
theta = x(11); 
psi   = x(12);
tao_u=ui(1);
tao_q=ui(2);
tao_r=ui(3);

% Get control inputs
% delta_s = -ui(2); 
% delta_r = ui(3);

% 45 degree maximum rudder angle
delta_max = 45 * pi/180;

% Check control inputs (useful later)
% if abs(delta_s) > delta_max && delta_s < delta_max
%     delta_s = sign(delta_s) * delta_max;
% end 
% 
% if abs(delta_r) > delta_max 
%     delta_r = sign(delta_r) * delta_max;
% end

% Initialize elements of coordinate system transform matrix
% ---------------------------------------- --------------------------------------
c1 = cos(phi); 
c2 = cos(theta); 
c3 = cos(psi); 
s1 = sin(phi); 
s2 = sin(theta); 
s3 = sin(psi); 
t2 = tan(theta);

% ----------------------------------------
% Vehicle Parameters and Coefficients
% ----------------------------------------
W = 2.99e2; % Weight (N)
B = 2.99e2; % Bouyancy (N)%% Note buoyanci incorrect simulation fail with this value

g = 9.81; % Force of gravity 
m = W/g; % Mass of vehicle

Xuu   = -1.62;    % Axial Drag
Xwq   = -3.55e1;  % Added mass cross-term
Xqq   = -1.93;    % Added mass cross-term
Xvr   =  3.55e1;  % Added mass cross-term
Xrr   = -1.93;    % Added mass cross-term
Yvv   = -1.31e3;  % Cross-flow drag
Yrr   =  6.32e-1; % Cross-flow drag
Yuv   = -2.86e1;  % Body lift force and fin lift
Ywp   =  3.55e1;  % Added mass cross-term
Yur   =  5.22;    % Added mass cross-term and fin lift
Ypq   =  1.93;    % Added mass cross-term
Zww   = -1.31e2;  % Cross-flow drag 
Zqq   = -6.32e-1; % Cross-flow drag
Zuw   = -2.86e1;  % Body lift force and fin lift
Zuq   = -5.22;    % Added mass cross-term and fin lift
Zvp   = -3.55e1;  % Added mass cross-term
Zrp   =  1.93;    % Added mass cross-term

% Center of Gravity wrt Origin at CB
xg = 0;
yg = 0;
zg = 1.96e-2;

% Control Fin Coefficients
Yuudr =  9.64;
Nuudr = -6.15;
Zuuds = -9.64; % Fin Lift Force

% Center of Buoyancy wrt Origin at Vehicle Nose
xb = 0;%-6.11e-1;
yb =  0;
zb =  0;
n=ui(1)/60*2*pi;
% Propeller Terms
Xprop =  1.569759e-4*n*abs(n);
Kpp   = -1.3e-1;  % Rolling resistance
Kprop = -2.242e-05*n*abs(n);%-5.43e-1; % Propeller Torque
Kpdot = -7.04e-2; % Added mass

% Cross flow drag and added mass terms
Mww   =  3.18; % Cross-flow drag
Mqq   = -1.88e2; % Cross-flow drag
Mrp   =  4.86; % Added mass cross-term
Muq   = -2; % Added mass cross term and fin lift
Muw   =  2.40e1; % Body and fin lift and munk moment
Mwdot = -1.93; % Added mass
Mvp   = -1.93; % Added mass cross term
Muuds = -6.15; % Fin lift moment
Nvv   = -3.18; % Cross-flow drag
Nrr   = -9.40e1; % Cross-flow drag
Nuv   = -2.40e1; % Body and fin lift and munk moment
Npq   = -4.86; % Added mass cross-term

% Moments of Inertia wrt Origin at CB
Ixx  = 1.77e-1;   
Iyy  = 3.45;  
Izz  = 3.45;

Nwp = -1.93; % Added mass cross-term
Nur = -2.00; % Added mass cross term and fin lift

% Non-linear Moments Coefficients
Xudot = -9.30e-1; % Added mass
Yvdot = -3.55e1;  % Added mass
Nvdot =  1.93;    % Added mass
Mwdot = -1.93;    % Added mass
Mqdot = -4.88;    % Added mass
Zqdot = -1.93;    % Added mass
Zwdot = -3.55e1;  % Added mass
Yrdot =  1.93;    % Added mass
Nrdot = -4.88;    % Added mass

% Set total forces from equations of motion
% ----------------------------------------------------- -------------------------
X = -(W-B)*sin(theta) + Xuu*u*abs(u) + (Xwq-m)*w*q + (Xqq + m*xg)*q^2 ...
    + (Xvr+m)*v*r + (Xrr + m*xg)*r^2 -m*yg*p*q - m*zg*p*r ...
    + Xprop ;

Y = (W-B)*cos(theta)*sin(phi) + Yvv*v*abs(v) + Yrr*r*abs(r) + Yuv*u*v ...
    + (Ywp+m)*w*p + (Yur-m)*u*r - (m*zg)*q*r + (Ypq - m*xg)*p*q ...
    + 0;%Yuudr*u^2*delta_r 

Z = (W-B)*cos(theta)*cos(phi) + Zww*w*abs(w) + Zqq*q*abs(q)+ Zuw*u*w ...
    + (Zuq+m)*u*q + (Zvp-m)*v*p + (m*zg)*p^2 + (m*zg)*q^2 ...
    + (Zrp - m*xg)*r*p  ;%+ Zuuds*u^2*delta_s

K = -(yg*W-yb*B)*cos(theta)*cos(phi) - (zg*W-zb*B)*cos(theta)*sin(phi) ...
    + Kpp*p*abs(p) - (Izz- Iyy)*q*r - (m*zg)*w*p + (m*zg)*u*r  ;%+ Kprop

M = -(zg*W-zb*B)*sin(theta) - (xg*W-xb*B)*cos(theta)*cos(phi) + Mww*w*abs(w) ...
    + Mqq*q*abs(q) + (Mrp - (Ixx-Izz))*r*p + (m*zg)*v*r - (m*zg)*w*q ...
    + (Muq - m*xg)*u*q + Muw*u*w + (Mvp + m*xg)*v*p ...
    + tao_q ;%Muuds*u^2*delta_s

N = -(xg*W-xb*B)*cos(theta)*sin(phi) - (yg*W-yb*B)*sin(theta) ...
    + Nvv*v*abs(v) + Nrr*r*abs(r) + Nuv*u*v ...
    + (Npq - (Iyy- Ixx))*p*q + (Nwp - m*xg)*w*p + (Nur + m*xg)*u*r ...
    + tao_r;% Nuudr*u^2*delta_r 


FORCES = [X Y Z K M N]';

% Accelerations Matrix (Prestero Thesis page 46)
Amat = [(m - Xudot) 0              0               0             m*zg            -m*yg;
        0           (m - Yvdot)    0               -m*zg         0               (m*xg - Yrdot);
        0           0              (m - Zwdot)     m*yg          (-m*xg - Zqdot) 0;
        0           -m*zg          m*yg            (Ixx - Kpdot) 0               0;
        m*zg        0              (-m*xg - Mwdot) 0             (Iyy - Mqdot)   0;
        -m*yg       (m*xg - Nvdot) 0               0             0               (Izz - Nrdot)];

% Inverse Mass Matrix
Minv = inv(Amat);

% Derivatives
xdot = ...
    [Minv(1,1)*X + Minv(1,2)*Y + Minv(1,3)*Z + Minv(1,4)*K + Minv(1,5)*M + Minv(1,6)*N
     Minv(2,1)*X + Minv(2,2)*Y + Minv(2,3)*Z + Minv(2,4)*K + Minv(2,5)*M + Minv(2,6)*N
     Minv(3,1)*X + Minv(3,2)*Y + Minv(3,3)*Z + Minv(3,4)*K + Minv(3,5)*M + Minv(3,6)*N
     Minv(4,1)*X + Minv(4,2)*Y + Minv(4,3)*Z + Minv(4,4)*K + Minv(4,5)*M + Minv(4,6)*N
     Minv(5,1)*X + Minv(5,2)*Y + Minv(5,3)*Z + Minv(5,4)*K + Minv(5,5)*M + Minv(5,6)*N
     Minv(6,1)*X + Minv(6,2)*Y + Minv(6,3)*Z + Minv(6,4)*K + Minv(6,5)*M + Minv(6,6)*N
     c3*c2*u + (c3*s2*s1-s3*c1)*v + (s3*s1+c3*c1*s2)*w
     s3*c2*u + (c1*c3+s1*s2*s3)*v + (c1*s2*s3-c3*s1)*w
       -s2*u +            c2*s1*v +            c1*c2*w
           p +            s1*t2*q +            c1*t2*r
                             c1*q -               s1*r
                          s1/c2*q +            c1/c2*r] ;
